simulink library "simlib_vpc_gp"  (R2022a)
settings: Solver=VariableStepAuto  StartTime=0.0  StopTime=10.0  RelTol=1e-3
undefined symbols (not defined in the file or in its folder): hyp_switchedGP1, M, Q, sn_switchedGP1, X_switchedGP1, Y_switchedGP1
settings Model: Creator=marco  LastModifiedBy=marco
settings SolverCC: AlgebraicLoopSolver=TrustRegion
settings DebuggingCC: UnconnectedInputMsg=warning  UnconnectedOutputMsg=warning  UnconnectedLineMsg=warning  SFMachineParentedDataDiag=warning
settings RTWCC: DLArmComputeVersion=19.05

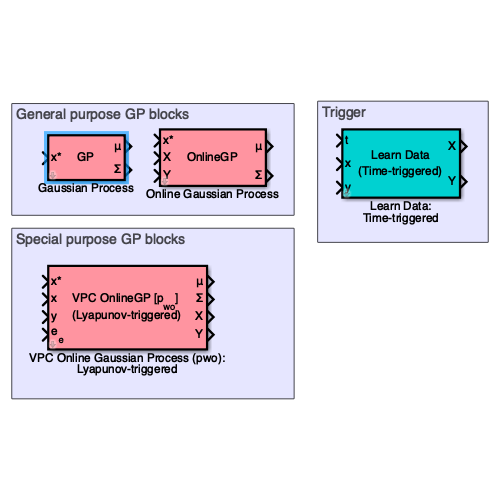
[thumbnail: Simulink's stored preview of the top-level diagram]
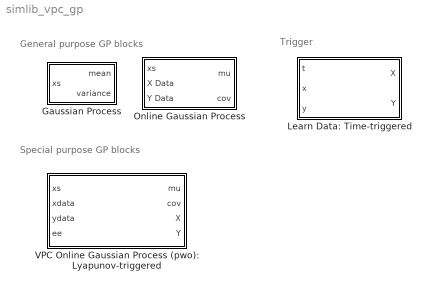
== system simlib_vpc_gp ==
  note: General purpose GP blocks
  note: Trigger
  note: Special purpose GP blocks
  Gaussian Process : Subsystem  TreatAsAtomicUnit=on  mask(Gaussian Process [V1]){X=X_switchedGP1, Y=Y_switchedGP1, sn=sn_switchedGP1, kernel=Squared Exponential ARD, hyp=hyp_switchedGP1, show_mean=on, show_variance=on, inv_fallback=on}
      mask prompts: X "Input X"; Y "Output Y"; sn "Noise standard deviation sn"; hyp "Hyperparameters"; show_mean "mean µ"; show_variance "variance ∑"; inv_fallback "Fallback: Inversion"
      mask help:
      | Gaussian Process Implementation based on mean-prior zero.
      |
      | Hyperparameters, I/O Data and kernel have to be set below.
      mask init:
      | %% Proof-check dimensions
      | 
      | % Process output flags
      | outport = 1;
      | if show_mean
      |     block = find_system(gcb,'SearchDepth','1','LookUnderMasks','on','FollowLinks','on','Name','Terminator_mean');
      |     try delete_line(gcb,'GP/1','Terminator_mean/1'); catch; end
      |     try delete_block(block); catch; end
      |     try add_block('built-in/Outport',[gcb,'/mean'],'Port',num2str(outport),'Position',[135 108 165 122]); catch; end
      |     try add_line(gcb,'GP/1','mean/1','autorouting','smart'); catch; end
      |     outport = outport + 1;
      | else
      |     block = find_system(gcb,'SearchDepth','1','LookUnderMasks','on','FollowLinks','on','Name','mean');
      |     try delete_line(gcb,'GP/1','mean/1'); catch; end
      |     try delete_block(block); catch; end
      |     try add_block('built-in/Terminator',[gcb,'/Terminator_mean'],'Position',[135 108 165 122]); catch; end
      |     try add_line(gcb,'GP/1','Terminator_mean/1','autorouting','smart'); catch; end
      | end
      | if show_variance
      |     block = find_system(gcb,'SearchDepth','1','LookUnderMasks','on','FollowLinks','on','Name','Terminator_variance');
      |     try delete_line(gcb,'GP/2','Terminator_variance/1'); catch; end
      |     try delete_block(block); catch; end
      |     try add_block('built-in/Outport',[gcb,'/variance'],'Port',num2str(outport),'Position',[135 148 165 162]); catch; end
      |     try add_line(gcb,'GP/2','variance/1','autorouting','smart'); catch; end
      |     outport = outport + 1;
      | else
      |     varianceblock = find_system(gcb,'SearchDepth','1','LookUnderMasks','on','FollowLinks','on','Name','variance');
      |     try delete_line(gcb,'GP/2','variance/1'); catch; end
      |     try delete_block(varianceblock); catch; end
      |     try add_block('built-in/Terminator',[gcb,'/Terminator_variance'],'Position',[135 148 165 162]); catch; end
      |     try add_line(gcb,'GP/2','Terminator_variance/1','autorouting','smart'); catch; end
      | end
      | 
      | % Check I/O Data dimensions
      | d = ndims(X);
      | if d == 3
      |     [N1,N2,M] = size(X);
      |     assert(N1==N2,'X does not seem to be pose data (at least not a 4x4xM matrix).');
      | else
      |     [M,N] = size(X);
      | end
      | [M_,Q_] = size(Y);
      | assert(M_==M,'Dimension mismatch! X & Y must have same number of data rows.');
      | if M == 0
      |     X = nan;
      |     Y = nan;
      | end
      | if ~isempty(sn)
      |     assert(isvector(sn),'Dimension mismatch! sigma_n must be a vector, not a matrix!');
      |     assert(length(sn)==Q_,'Dimension mismatch! Define noise variance for every output y! sigma_n:[1:%i] ~= Y:[*:%i]',length(sn),size(Y,2));
      | else
      |     sn = nan;
      | end
      | 
      | % Check kernel hyperparameter dimensions
      | [Q,n] = size(hyp);
      | assert(Q > 0 && n > 0, 'kernel hyperparameters cannot be empty');
      | switch kernel
      |     case {1,3,5,6} %'SE', 'Matern' or 'SE3'
      |         if kernel == 1
      |             kernelfun = @SE;
      |         elseif kernel == 3
      |             kernelfun = @Matern;
      |         elseif kernel == 5
      |             kernelfun = @SE3Axang;
      |         elseif kernel == 6
      |             kernelfun = @SE3Hom;
      |         end
      |         if Q_ > 0
      |             assert(Q==Q_,'Mismatch in kernel hyperparameters! hyp:[%i,:]~=[%i,:]',Q,Q_);
      |         end
      |         assert(n==2,'Mismatch in kernel hyperparameters! hyp:[:,%i]~=[:,%i]',n,2);
      |     case {2,4} %'SEARD' or 'MaternARD'
      |         if kernel == 2
      |             kernelfun = @SEARD;
      |         else
      |             kernelfun = @MaternARD;
      |         end
      |         if Q_ ~= 0
      |             assert(n==N+1 & Q==Q_,'Mismatch in kernel hyperparameters! hyp:[%i,%i]~=[%i,%i]',Q,n,Q_,N+1);
      |         end
      |         if N > 0
      |             assert(n==N+1,'Mismatch in kernel hyperparameters! hyp:[:,%i]~=[:,%i]',n,N+1);
      |         end
      |     otherwise
      |         error('Kernel not supported');
      | end
      mask Help:
      | Refer to:
      | C. E. Rasmussen and C. K. I. Williams, <i>Gaussian Processes for Machine Learning</i>. MIT Press, 2006.
      mask TypeOptions kernel: Squared Exponential | Squared Exponential ARD | Matern | Matern ARD | SE3 (Axis-Angle) | SE3 (Homogeneous)
      mask DialogControl DataGroupVar Prompt: I/O Data
      mask DialogControl X Tooltip: Dimensions: M x N
      mask DialogControl Y Tooltip: Dimensions: M x Q
      mask DialogControl sn Tooltip: Dimensions: Q
      mask DialogControl KernelGroupVar Prompt: Kernel Parameters
      mask DialogControl hyp Tooltip: Dimensions: Q * (kernel length)
      mask DialogControl OutputGroupVar Prompt: Show outputs
      mask DialogControl inv_fallback Tooltip: If checked, uses the standard inversion inv(K) for the kernel matrix K.
      mask Display:
      | % Write label
      | disp('GP','texmode','on')
      | 
      | % Label ports
      | outport = 1;
      | port_label('input',1,'x*','texmode','on')
      | if strcmp(get_param(gcb,"show_mean"),'on')
      |     port_label('output',outport,'\mu','texmode','on')
      |     outport = outport + 1;
      | end
      | if strcmp(get_param(gcb,"show_variance"),'on')
      |     port_label('output',outport,'\Sigma','texmode','on')
      |     outport = outport + 1;
      | end
  Learn Data: Time-triggered : Subsystem  TreatAsAtomicUnit=on  mask(Time-triggered Learning [V1]){ts=0.01, T=1, M=10, forget_type=oldest}
      mask prompts: ts "Sample time"; T "Trigger after (seconds)"; M "Maximum Datapoints"; forget_type "Discard datapoint"
      mask help:
      | Learns Data that is passed to the block and outputs them as X & Y matrices (signals are variable-size!).
      |
      | Please note:
      | The maximum number of datapoints is limited as 100.
      | If you need more datapoints, you can fork this block by disabling the library link and then:
      | - alter the bounds for the variable size signal in the "Edit Data" panel of the Matlab Function block inside this block
      | - remove or change the mask Parameters & Dialogue pannel code at the corresponding line
      mask init:
      | % Check if all values are valid
      | 
      | assert(mod(T,ts)==0,'Trigger time must be a multiple of sample time!');
      mask TypeOptions ts: Rate Transition/OutPortSampleTime | Rate Transition1/OutPortSampleTime | Rate Transition2/OutPortSampleTime
      mask TypeOptions forget_type: oldest | newest
      mask DialogControl T Tooltip: Needs to be a multiple of the sample time
      mask DialogControl forget_type Tooltip: When maximum number of datapoints has been reached, this rule decides what to do with the data
      mask Display:
      | % Write label
      | disp(["    Learn Data"; "(Time-triggered)"],'texmode','on')
      | 
      | % Label ports
      | port_label('input',1,'t','texmode','on')
      | port_label('input',2,'x','texmode','on')
      | port_label('input',3,'y','texmode','on')
      | port_label('output',1,'X','texmode','on')
      | port_label('output',2,'Y','texmode','on')
  Online Gaussian Process : Subsystem  TreatAsAtomicUnit=on  mask(Online Gaussian Process [V1]){sn_source=internal, sn=[], kernel=Squared Exponential ARD, hyp_source=internal, hyp=[]}
      mask prompts: sn_source "Noise source"; sn "Noise standard variation sn"; hyp_source "Hyperparameter source"; hyp "Hyperparameters"
      mask help:
      | Online Gaussian Process Implementation based on mean-prior zero.
      |
      | Hyperparameters, noise and kernel have to be set below.
      mask init:
      | %% Switch input source
      | portnum = 4;
      | 
      | % Switch: hyp source
      | block = find_system(gcb,'SearchDepth','1','LookUnderMasks','on',...
      |     'FollowLinks','on','Name','hyp');
      | try; delete_line(gcb,'hyp/1','OnlineGP/4'); end;
      | try; delete_block(block); end;
      | switch hyp_source
      |     case 1 % Make internal
      |         try; add_block('built-in/Constant',[gcb,'/hyp'],'Value','hyp','Position',[-90 175 -70 195]); end;
      |     case 2 % Make external
      |         try; add_block('built-in/Inport',[gcb,'/hyp'],'Position',[-95 178 -65 192],'Port',num2str(portnum)); end;
      |         portnum = portnum + 1;
      | end
      | try; add_line(gcb,'hyp/1','OnlineGP/4','autorouting','smart'); end;
      | 
      | % Switch: sn source
      | block = find_system(gcb,'SearchDepth','1','LookUnderMasks','on',...
      |     'FollowLinks','on','Name','sn');
      | try; delete_line(gcb,'sn/1','OnlineGP/5'); end;
      | try; delete_block(block); end;
      | switch sn_source
      |     case 1 % Make internal
      |         try; add_block('built-in/Constant',[gcb,'/sn'],'Value','sn','Position',[-85 202 -70 218]); end;
      |     case 2 % Make external
      |         try; add_block('built-in/Inport',[gcb,'/sn'],'Position',[-95 203 -65 217],'Port',num2str(portnum)); end;
      |         portnum = portnum + 1;
      | end
      | try; add_line(gcb,'sn/1','OnlineGP/5','autorouting','smart'); end;
      | 
      | 
      | %% Proof-check dimensions
      | if strcmp(sn_source,'internal')
      |     % Check I/O Data dimensions
      |     if ~isempty(sn)
      |         assert(isvector(sn),'Dimension mismatch! sigma_n must be a vector, not a matrix!');
      |     end
      |     Q = length(sn);
      | 
      |     % Check kernel hyperparameter dimensions
      |     [q,n] = size(hyp);
      |     switch kernel
      |         case 1 %'SE'
      |             %kernelfun = @SE;
      |             if strcmp(hyp_source,'internal')
      |                 if ~isempty(hyp)
      |                     assert(n==2 & q==Q,'Mismatch in kernel hyperparameters! hyp:[%i,%i]~=[%i,2]',q,n,Q,2);
      |                 end
      |             end
      |         case 2 %'SEARD'
      |             %kernelfun = @SEARD;
      |         otherwise
      |             error('Kernel not supported');
      |     end
      | end
      mask Help:
      | Refer to:
      | C. E. Rasmussen and C. K. I. Williams, <i>Gaussian Processes for Machine Learning</i>. MIT Press, 2006.
      mask TypeOptions sn_source: internal | external
      mask Callback sn_source:
      | idx = find(strcmp(get_param(gcb,'MaskNames'),'sn'));
      | maskvis = get_param(gcb,'MaskVisibilities');
      | switch get_param(gcb,'sn_source')
      |     case 'internal' % Show field
      |         maskvis{idx} = 'on';
      |     case 'external' % Hide field
      |         maskvis{idx} = 'off';
      | end
      | set_param(gcb,'MaskVisibilities',maskvis);
      mask TypeOptions kernel: Squared Exponential | Squared Exponential ARD
      mask TypeOptions hyp_source: internal | external
      mask Callback hyp_source:
      | idx = find(strcmp(get_param(gcb,'MaskNames'),'hyp'));
      | maskvis = get_param(gcb,'MaskVisibilities');
      | switch get_param(gcb,'hyp_source')
      |     case 'internal' % Show field
      |         maskvis{idx} = 'on';
      |     case 'external' % Hide field
      |         maskvis{idx} = 'off';
      | end
      | set_param(gcb,'MaskVisibilities',maskvis);
      mask DialogControl DataGroupVar Prompt: I/O Data
      mask DialogControl sn Tooltip: Dimensions: Q
      mask DialogControl KernelGroupVar Prompt: Kernel Parameters
      mask DialogControl hyp Tooltip: Dimensions: Q * (kernel length)
      mask Display:
      | % Write label
      | disp('OnlineGP','texmode','on')
      | 
      | % Label ports
      | portnum = 4;
      | port_label('input',1,'x*','texmode','on')
      | port_label('input',2,'X','texmode','on')
      | port_label('input',3,'Y','texmode','on')
      | if strcmp(get_param(gcb,'hyp_source'),'external')
      |     port_label('input',portnum,'hyp','texmode','on')
      |     portnum = portnum + 1;
      | end
      | if strcmp(get_param(gcb,'sn_source'),'external')
      |     port_label('input',portnum,'sn','texmode','on')
      |     portnum = portnum + 1;
      | end
      | port_label('output',1,'\mu','texmode','on')
      | port_label('output',2,'\Sigma','texmode','on')
  VPC Online Gaussian Process (pwo): Lyapunov-triggered : Subsystem  TreatAsAtomicUnit=on  mask(VPC Online Gaussian Process (Lyapunov-triggered, pwo) [V1]){M=10, Xinit=nan, Yinit=nan, sn=[], kernel=Squared Exponential ARD, hyp=[], optimize=off, ts=0.01, lambda=1, beta=[], forget_type=oldest}
      mask prompts: M "Maximum Datapoints"; Xinit "Initial input X"; Yinit "Initial output Y"; sn "Initial noise variance"; hyp "Initial hyperparameters"; optimize "Optimize Hyperparameters online"; ts "Sample time"; lambda "Lambda λ_Q"; beta "Beta β"; forget_type "Discard datapoint"
      mask help:
      | Specialized Online Gaussian Process implementation for VPC based on mean-prior zero and a Lyapunov-Trigger.
      | The Lyapunov trigger is:
      | Δf ≥ λ_Q ||e_e||    with Δf=βΣ(p_wo)
      |
      | Note 1:
      | - x* is the input to evaluate the GP model for.
      | - x and y are the data to be learned if a trigger event occurs
      | The special distinction between x* and x is due to how the Simulink and the sample time of blocks with persistent variables work, but it can also be used to test the influence of noise.
      |
      | Note 2:
      | The maximum number of datapoints is limited as 100.
      | If you need more datapoints, you can fork this block by disabling the library link and then:
      | - alter the bounds for the variable size signal in the "Edit Data" panel of the Matlab Function block inside this block
      | - remove or change the mask Parameters & Dialogue pannel code at the corresponding line
      mask init:
      | %% Proof-check dimensions
      | 
      | % Check I/O Data dimensions
      | if ~isnan(Xinit)
      |     assert(size(Xinit,1)==M,'Dimension mismatch! X must have same number of data rows.');
      | end
      | if ~isnan(Yinit)
      |     assert(size(Yinit,1)==M,'Dimension mismatch! Y must have same number of data rows.');
      | end
      | Q = length(sn);
      | if ~isempty(sn)
      |     assert(isvector(sn),'Dimension mismatch! sigma_n must be a vector, not a matrix!');
      |     assert(Q==6,'Dimension mismatch! Define noise variance for every output y (there are 6!). sigma_n:[1:%i] ~= [1:6]',Q);
      | end
      | 
      | % Check kernel hyperparameter dimensions
      | [q,n] = size(hyp);
      | switch kernel
      |     case 1 %'SE'
      |         kernelfun = @SE;
      |         if ~isempty(hyp)
      |             assert(n==2 & q==Q,'Mismatch in kernel hyperparameters! hyp:[%i,%i]~=[%i,2]',q,n,Q,2);
      |         end
      |     case 2 %'SEARD'
      |         kernelfun = @SEARD;
      |         if ~isempty(hyp)
      |             assert(n==4 & q==Q,'Mismatch in kernel hyperparameters! hyp:[%i,%i]~=[%i,4]',q,n,Q);
      |         end
      |     otherwise
      |         error('Kernel not supported');
      | end
      | 
      | % Check beta
      | if ~isempty(beta)
      |     assert(isvector(beta) && length(beta)==Q,'Mismatch in beta dimensions! beta:[1:%i]~=[1,%i]',length(beta),Q);
      | end
      mask Help:
      | Refer to:
      | C. E. Rasmussen and C. K. I. Williams, <i>Gaussian Processes for Machine Learning</i>. MIT Press, 2006.
      mask TypeOptions kernel: Squared Exponential | Squared Exponential ARD
      mask TypeOptions ts: Rate Transition1/OutPortSampleTime | Rate Transition2/OutPortSampleTime | Rate Transition3/OutPortSampleTime
      mask TypeOptions forget_type: oldest | newest | optimize
      mask DialogControl DataGroupVar Prompt: I/O Data
      mask DialogControl Xinit Tooltip: Dimensions: M x N. Specifiying "nan" means to not provide data.
      mask DialogControl Yinit Tooltip: Dimensions: M x Q. Specifiying "nan" means to not provide data.
      mask DialogControl sn Tooltip: Dimensions: Q
      mask DialogControl KernelGroupVar Prompt: Kernel Parameters
      mask DialogControl hyp Tooltip: Dimensions: Q * (kernel length)
      mask DialogControl TriggerGroupVar Prompt: Trigger Parameters
      mask Display:
      | % Write label
      | disp(["VPC OnlineGP [p_{wo}]";"(Lyapunov-triggered)"],'texmode','on')
      | 
      | % Label ports
      | port_label('input',1,'x*','texmode','on')
      | port_label('input',2,'x','texmode','on')
      | port_label('input',3,'y','texmode','on')
      | port_label('input',4,'e_e','texmode','on')
      | port_label('output',1,'\mu','texmode','on')
      | port_label('output',2,'\Sigma','texmode','on')
      | port_label('output',3,'X','texmode','on')
      | port_label('output',4,'Y','texmode','on')

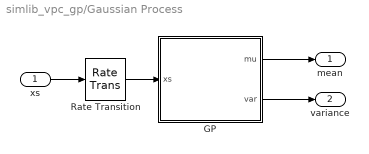
== system simlib_vpc_gp/Gaussian Process ==
  xs : Inport
  GP : MATLAB Function  TreatAsAtomicUnit=on
  Rate Transition : RateTransition
  mean : Outport
  variance : Outport  Port=2
  wires:
  GP/2(var) -> variance/1
  Rate Transition/1 -> GP/1(xs)
  xs/1 -> Rate Transition/1
  GP/1(mu) -> mean/1

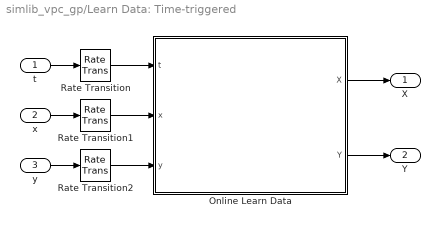
== system simlib_vpc_gp/Learn Data: Time-triggered ==
  t : Inport
  x : Inport  Port=2
  y : Inport  Port=3
  Online Learn Data : MATLAB Function  TreatAsAtomicUnit=on
  Rate Transition : RateTransition  OutPortSampleTime=ts
  Rate Transition1 : RateTransition  OutPortSampleTime=ts
  Rate Transition2 : RateTransition  OutPortSampleTime=ts
  X : Outport
  Y : Outport  Port=2
  wires:
  Rate Transition/1 -> Online Learn Data/1(t)
  Rate Transition1/1 -> Online Learn Data/2(x)
  Rate Transition2/1 -> Online Learn Data/3(y)
  t/1 -> Rate Transition/1
  x/1 -> Rate Transition1/1
  y/1 -> Rate Transition2/1
  Online Learn Data/1(X) -> X/1
  Online Learn Data/2(Y) -> Y/1

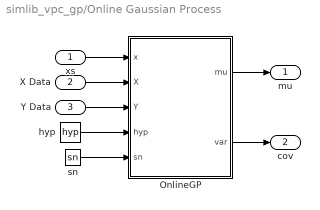
== system simlib_vpc_gp/Online Gaussian Process ==
  xs : Inport
  X Data : Inport  Port=2
  Y Data : Inport  Port=3
  OnlineGP : MATLAB Function  TreatAsAtomicUnit=on
  hyp : Constant  Value=hyp
  sn : Constant  Value=sn
  mu : Outport
  cov : Outport  Port=2
  wires:
  OnlineGP/1(mu) -> mu/1
  OnlineGP/2(var) -> cov/1
  xs/1 -> OnlineGP/1(x)
  X Data/1 -> OnlineGP/2(X)
  Y Data/1 -> OnlineGP/3(Y)
  hyp/1 -> OnlineGP/4(hyp)
  sn/1 -> OnlineGP/5(sn)

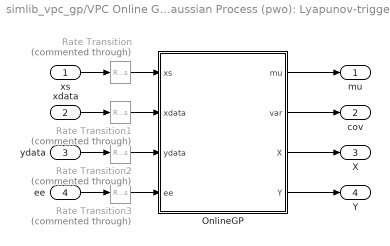
== system simlib_vpc_gp/VPC Online Gaussian Process (pwo): Lyapunov-triggered ==
  xs : Inport
  xdata : Inport  Port=2
  ydata : Inport  Port=3
  ee : Inport  Port=4
  OnlineGP : MATLAB Function  TreatAsAtomicUnit=on
  Rate Transition : RateTransition  Commented=through
  Rate Transition1 : RateTransition  Commented=through  OutPortSampleTime=ts
  Rate Transition2 : RateTransition  Commented=through  OutPortSampleTime=ts
  Rate Transition3 : RateTransition  Commented=through  OutPortSampleTime=ts
  mu : Outport
  cov : Outport  Port=2
  X : Outport  Port=3
  Y : Outport  Port=4
  wires:
  xs/1 -> Rate Transition/1
  OnlineGP/2(var) -> cov/1
  OnlineGP/1(mu) -> mu/1
  ydata/1 -> Rate Transition2/1
  ee/1 -> Rate Transition3/1
  OnlineGP/3(X) -> X/1
  OnlineGP/4(Y) -> Y/1
  xdata/1 -> Rate Transition1/1
  Rate Transition/1 -> OnlineGP/1(xs)
  Rate Transition1/1 -> OnlineGP/2(xdata)
  Rate Transition2/1 -> OnlineGP/3(ydata)
  Rate Transition3/1 -> OnlineGP/4(ee)

== matlab function simlib_vpc_gp/Learn Data: Time-triggered/Online Learn Data ==
  data: X output size=[100 6]; t input; Y output size=[100 6]; x input; y input; M parameter; T parameter; forget_type parameter
function [X,Y] = onlinelearn_timetriggered(t,x,y,M,T,forget_type) %#codegen
%%ONLINELEARN_TIMETRIGGERED learns new datapoint by a time-trigger
%
% Editor:
%   OMAINSKA Marco - Doctoral Student, Cybernetics
%       <marcoomainska@g.ecc.u-tokyo.ac.jp>
% Review:
%   YAMAUCHI Junya - Assistant Professor
%       <junya_yamauchi@ipc.i.u-tokyo.ac.jp>
%
% Property of: Fujita-Yamauchi Lab, University of Tokyo, 2021
% e-mail: marcoomainska@g.ecc.u-tokyo.ac.jp
% Website: https://www.scl.ipc.i.u-tokyo.ac.jp
% January 2022
%
%------------- BEGIN CODE --------------

N = length(x);

% define persistent data
persistent X_ Y_
coder.varsize('X_',[M N])
coder.varsize('Y_',[M N])

% init data
if isempty(X_) || isempty(Y_)
    X_ = zeros(0,N);
    Y_ = zeros(0,N);
end

% append datapoint if triggered
if M > 0
    if mod(t,T) == 0 % trigger
        if size(X_,1) < M
            % Learn new datapoint
            X_ = [X_; x(:)'];
            Y_ = [Y_; y(:)'];
        else
            % Forget datapoint
            switch forget_type
                case 1 %'oldest'
                    % Discard oldest
                    X_ = [X_(2:M,:); x(:)'];
                    Y_ = [Y_(2:M,:); y(:)'];
                case 2 %'newest'
                    % Discard newest -> nothing to do
                otherwise
                    error('Unknown forget rule');
            end
        end
    end
end

% set output
X = X_;
Y = Y_;

end

== matlab function simlib_vpc_gp/Gaussian Process/GP ==
  data: xs input; mu output; var output; X parameter; Y parameter; kernel parameter size=1; hyp parameter; sn parameter; M parameter size=1; Q parameter size=1; inv_fallback parameter size=1
function [mu, var] = gp_slx(xs, X, Y, kernel, hyp, sn, M, Q, inv_fallback) %#codegen
% Function Wrapper
%
% Editor:
%   OMAINSKA Marco - Doctoral Student, Cybernetics
%       <marcoomainska@g.ecc.u-tokyo.ac.jp>
% Review:
%   YAMAUCHI Junya - Assistant Professor
%       <junya_yamauchi@ipc.i.u-tokyo.ac.jp>
%
% Property of: Fujita-Yamauchi Lab, University of Tokyo, 2021
% e-mail: marcoomainska@g.ecc.u-tokyo.ac.jp
% Website: https://www.scl.ipc.i.u-tokyo.ac.jp
% April 2021
%
%------------- BEGIN CODE --------------
persistent Kinv A

% define kernel-function
switch kernel
    case 1 %'SE'
        kernelfun = @SE;
        xs_ = xs(:)';
    case 2 %'SEARD'
        kernelfun = @SEARD;
        xs_ = xs(:)';
    case 3 %'Matern'
        kernelfun = @Matern;
        xs_ = xs(:)';
    case 4 %'MaternARD'
        kernelfun = @MaternARD;
        xs_ = xs(:)';
    case 5 %'SE3 (Axis-Angle)'
        kernelfun = @SE3Axang;
        xs_ = xs(:)';
    case 6 %'SE3 (Homogeneous)'
        kernelfun = @SE3Hom;
        xs_ = xs;
    otherwise
        error('Kernel not supported');
end

% init inverse K and A matrices if not yet initialized
if isempty(Kinv) || isempty(A)
    if M > 0 && Q > 0
        Kinv = zeros(M,M,Q);
        A = zeros(M,Q);
        for q=1:Q
            K = kernelfun(X,X,hyp(q,:)) + sn(q)^2*eye(M);
            if ~inv_fallback % try cholesky, else do fallback to normal matrix inversion
                L = chol(K,"lower"); % A = L*L'
                Kinv(:,:,q) = (L\eye(M))'*(L\eye(M)); % A^-1 = L^-T*L^-1
                %Kinv(:,:,q) = inv(L)'*inv(L); % A^-1 = L^-T*L^-1
            else
                Kinv(:,:,q) = inv(K);
            end
            A(:,q) = Kinv(:,:,q) * Y(:,q);
        end
        % A = pagemtimes(Kinv,Y); % not supported by MATLAB codegen
    else
        Kinv = nan; A = nan;
    end
end

% calculate GP output
%   Note: "gp_calc" is a MATLAB function on the MATLAB path
if M > 0
    [mu_, var_] = gp_calc(xs_, X, Y, kernelfun, hyp, sn, Kinv, A);
else
    [mu_, var_] = gp_calc(xs_, [], [], kernelfun, hyp, sn, [], []);
end
mu = mu_'; var = var_';

%-------------- END CODE ---------------
end

== matlab function simlib_vpc_gp/Online Gaussian Process/OnlineGP ==
  data: x input; mu output; var output; kernel parameter size=1; X input; Y input; hyp input; sn input
function [mu, var] = onlinegp_slx(x, kernel, X, Y, hyp, sn) %#codegen
% Function Wrapper
%
% Editor:
%   OMAINSKA Marco - Doctoral Student, Cybernetics
%       <marcoomainska@g.ecc.u-tokyo.ac.jp>
% Review:
%   YAMAUCHI Junya - Assistant Professor
%       <junya_yamauchi@ipc.i.u-tokyo.ac.jp>
%
% Property of: Fujita-Yamauchi Lab, University of Tokyo, 2021
% e-mail: marcoomainska@g.ecc.u-tokyo.ac.jp
% Website: https://www.scl.ipc.i.u-tokyo.ac.jp
% January 2022
%
%------------- BEGIN CODE --------------
persistent Kinv A X_ Y_
coder.varsize('Kinv');
coder.varsize('A');

% preprocess inputs
xs = x(:)';

% output dimension
Q = length(sn);

% init internal copy of I/O Data if not yet initialized
if isempty(X_) || isempty(Y_)
    X_ = X; Y_ = Y;
end

% update internal copies of data if they have changed
if ~isequal(X_,X) || ~isequal(Y_,Y)
    X_ = X; Y_ = Y;
    
    % clear Kinv and A
    A = zeros(0,Q);
    Kinv = zeros(0,0,Q);
end

% calculate output
mu = zeros(Q,1);
var = zeros(Q,1);
if ~isempty(X_) && ~isempty(Y_)
    % define kernel-function
    switch kernel
        case 1 %'SE'
            kernelfun = @SE;
        case 2 %'SEARD'
            kernelfun = @SEARD;
        otherwise
            error('Kernel not supported');
    end
    
    % init inverse K and A matrices if not yet initialized
    M = size(X_,1);
    if isempty(Kinv) || isempty(A)
        A = zeros(M,Q);
        Kinv = zeros(M,M,Q);
        for q=1:Q
            L = chol(kernelfun(X,X,hyp(q,:)) + sn(q)^2*eye(M),"lower"); % A = L*L'
            Kinv(:,:,q) = (L\eye(M))'*(L\eye(M)); % A^-1 = L^-T*L^-1
            %Kinv(:,:,q) = inv(L)'*inv(L); % A^-1 = L^-T*L^-1
            %Kinv(:,:,q) = inv(kernelfun(X,X,hyp(q,:)) + sn(q)^2*eye(M));
            A(:,q) = Kinv(:,:,q) * Y(:,q);
        end
        % A = pagemtimes(Kinv,Y); % not supported by MATLAB codegen
    end

    % calculate GP output
    %   Note: "gp_calc" is a MATLAB function on the MATLAB path
    [mu_, var_] = gp_calc(x, X, Y, kernelfun, hyp, sn, Kinv, A);
    mu = mu_'; var = var_';
end

%-------------- END CODE ---------------
end

== matlab function simlib_vpc_gp/VPC Online Gaussian Process (pwo): Lyapunov-triggered/OnlineGP ==
  data: xs input; xdata input; ydata input; ee input; M parameter; mu output; var output; Xinit parameter; Yinit parameter; kernel parameter size=1; hyp parameter; sn parameter; X output size=[100,3]; Y output size=[100,6]; lambda parameter; beta parameter; forget_type parameter; optimize parameter
function [mu, var, X, Y] = onlinegp_slx(xs,xdata,ydata,ee,M,Xinit,Yinit,kernel,hyp,sn,lambda,beta,forget_type,optimize) %#codegen
% Function Wrapper
%
% Editor:
%   OMAINSKA Marco - Doctoral Student, Cybernetics
%       <marcoomainska@g.ecc.u-tokyo.ac.jp>
% Review:
%   YAMAUCHI Junya - Assistant Professor
%       <junya_yamauchi@ipc.i.u-tokyo.ac.jp>
%
% Property of: Fujita-Yamauchi Lab, University of Tokyo, 2022
% e-mail: marcoomainska@g.ecc.u-tokyo.ac.jp
% Website: https://www.scl.ipc.i.u-tokyo.ac.jp
% January 2022
%
%------------- BEGIN CODE --------------

% preprocess inputs
xs = xs(:)';
xdata = xdata(:)';
ydata = ydata(:)';

% dimensions
N = length(xs);
Q = length(sn);

% define kernel-function
switch kernel
    case 1 %'SE'
        kernelfun = @SE;
    case 2 %'SEARD'
        kernelfun = @SEARD;
    otherwise
        error('Kernel not supported');
end

% persistent variables
persistent X_ Y_ A Kinv
coder.varsize('X_',[M N]);
coder.varsize('Y_',[M Q]);
coder.varsize('A',[M Q]);
coder.varsize('Kinv',[M M Q]);

% init internal copy of I/O Data if not yet initialized
if isempty(X_) || isempty(Y_)
    if isnan(Xinit) || isnan(Yinit)
        X_ = zeros(0,N); Y_ = zeros(0,Q);
    else
        X_ = Xinit; Y_ = Yinit;
    end
    A = zeros(0,Q);
    Kinv = zeros(0,0,Q);
end

% Learn Dataset
if M > 0
    Deltaf = model_error(xdata,X_,Y_,kernelfun,hyp,sn,Kinv,A,beta);
    
    % check trigger
    % TODO: make trigger for outside noise set
    if Deltaf >= lambda*norm(ee,2)
        if size(X_,1) < M
            % Learn new datapoint
            X_ = [X_; xdata(:)'];
            Y_ = [Y_; ydata(:)'];
        else
            % Forget datapoint
            switch forget_type
                case 1 %'oldest'
                    % Discard oldest
                    X_ = [X_(2:M,:); xdata(:)'];
                    Y_ = [Y_(2:M,:); ydata(:)'];
                case 2 %'newest'
                    % Discard newest -> nothing to do
                case 3 %'optimize'
                    error('Not yet implemented');
                otherwise
                    error('Unknown forget rule');
            end
        end
        
        % Optimize Hyperparameters
        if optimize
            % TODO: Implement
        end
        
        % clear Kinv and A
        A = zeros(0,Q);
        Kinv = zeros(0,0,Q);
    end
end

% calculate output
mu = zeros(Q,1);
var = zeros(Q,1);
X = X_;
Y = Y_;
if ~isempty(X_) && ~isempty(Y_)
    % init inverse K and A matrices if not yet initialized
    M_ = size(X_,1);
    if isempty(Kinv) || isempty(A)
        A = zeros(M_,Q);
        Kinv = zeros(M_,M_,Q);
        for q=1:Q
            L = chol(kernelfun(X,X,hyp(q,:)) + sn(q)^2*eye(M),"lower"); % A = L*L'
            Kinv(:,:,q) = (L\eye(M))'*(L\eye(M)); % A^-1 = L^-T*L^-1
            %Kinv(:,:,q) = inv(L)'*inv(L); % A^-1 = L^-T*L^-1
            %Kinv(:,:,q) = inv(kernelfun(X_,X_,hyp(q,:)) + sn(q)^2*eye(M_));
            A(:,q) = Kinv(:,:,q) * Y_(:,q);
        end
        % A = pagemtimes(Kinv,Y); % not supported by MATLAB codegen
    end

    % calculate GP output
    %   Note: "gp_calc" is a MATLAB function on the MATLAB path
    [mu_, var_] = gp_calc(xs, X_, Y_, kernelfun, hyp, sn, Kinv, A);
    mu = mu_'; var = var_';
end

%-------------- END CODE ---------------
end


function Deltaf = model_error(x,X,Y,kernelfun,hyp,sn,Kinv,A,beta)
%%MODEL_ERROR returns model error Deltaf
%
% Editor:
%   OMAINSKA Marco - Doctoral Student, Cybernetics
%       <marcoomainska@g.ecc.u-tokyo.ac.jp>
% Review:
%   YAMAUCHI Junya - Assistant Professor
%       <junya_yamauchi@ipc.i.u-tokyo.ac.jp>
%
% Property of: Fujita-Yamauchi Lab, University of Tokyo, 2021
% e-mail: marcoomainska@g.ecc.u-tokyo.ac.jp
% Website: https://www.scl.ipc.i.u-tokyo.ac.jp
% January 2022
%
%------------- BEGIN CODE --------------

% Default: If there is no data yet, then the model error is infinity
if isempty(X) || isempty(Y)
    Deltaf = inf;
    return
end

% Sigma
%   Note: "gp_calc" is a MATLAB function on the MATLAB path
[~, var] = gp_calc(x, X, Y, kernelfun, hyp, sn, Kinv, A);

% Model error: Deltaf = ||beta^T*Sigma^{1/2}||
Deltaf = norm(dot(beta,sqrt(var)),2);

end
